simulink model "DCmotor"  (R2016a)
settings: Solver=ode23t  StartTime=0.0  StopTime=10.0  RelTol=1e-3  AbsTol=1e-3
libraries: fl_lib x12, nesl_utility x4
settings Model: Creator=STF2972  LastModifiedBy=STF2972
settings GRTTargetCC: GeneratePreprocessorConditionals=Use local settings
settings SimscapeCC: SimscapeLogType=all  SimscapeLogDataHistory=10000

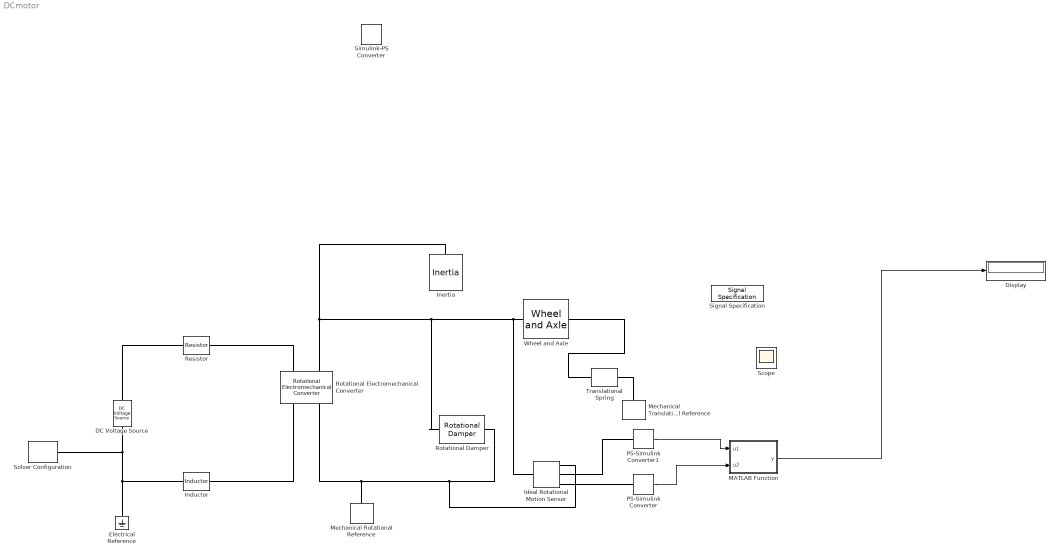
== system DCmotor ==
  DC Voltage Source : fl_lib/Electrical/Electrical Sources/DC Voltage Source  v0=5 V
  Display : Display
  Electrical Reference : fl_lib/Electrical/Electrical Elements/Electrical Reference
  Ideal Rotational Motion Sensor : fl_lib/Mechanical/Mechanical Sensors/Ideal Rotational Motion Sensor  offset=0 rad
  Inductor : fl_lib/Electrical/Electrical Elements/Inductor  l=1e-6 H  r=0 Ohm  g=1e-9 1/Ohm  i_specify=off  i_priority=None  i=0 A  v_specify=off  v_priority=None  v=0 V  i_L_specify=off  i_L_priority=High  i_L=0 A
  Inertia : fl_lib/Mechanical/Rotational Elements/Inertia  inertia=0.01 kg*m^2  w_specify=off  w_priority=High  w=0 rad/s  t_specify=off  t_priority=None  t=0 N*m
  MATLAB Function : MATLAB Function  TreatAsAtomicUnit=on
  Mechanical Rotational Reference : fl_lib/Mechanical/Rotational Elements/Mechanical Rotational Reference
  Mechanical Translational Reference : fl_lib/Mechanical/Translational Elements/Mechanical Translational Reference
  PS-Simulink Converter : nesl_utility/PS-Simulink Converter  PhysicalDomain=network_engine_domain  SubClassName=ps_output  LeftPortType=input  RightPortType=output  PseudoPeriodic=off  Frequencies=[]  Unit=deg  AffineConversion=off
  PS-Simulink Converter1 : nesl_utility/PS-Simulink Converter  PhysicalDomain=network_engine_domain  SubClassName=ps_output  LeftPortType=input  RightPortType=output  PseudoPeriodic=off  Frequencies=[]  Unit=1  AffineConversion=off
  Resistor : fl_lib/Electrical/Electrical Elements/Resistor  R=1 Ohm  i_specify=off  i_priority=None  i=0 A  v_specify=off  v_priority=None  v=0 V
  Rotational Electromechanical Converter : fl_lib/Electrical/Electrical Elements/Rotational Electromechanical Converter  K=0.1 V/(rad/s)  i_specify=off  i_priority=None  i=0 A  v_specify=off  v_priority=None  v=0 V  t_specify=off  t_priority=None  t=0 N*m  w_specify=off  w_priority=None  w=0 rad/s
  Rotational Damper : fl_lib/Mechanical/Rotational Elements/Rotational Damper  D=0.001 N*m/(rad/s)  w_specify=off  w_priority=None  w=0 rad/s  t_specify=off  t_priority=None  t=0 N*m
  Scope : Scope
  Signal Specification : SignalSpecification
  Simulink-PS Converter : nesl_utility/Simulink-PS Converter  PhysicalDomain=network_engine_domain  SubClassName=ps_input  LeftPortType=input  RightPortType=output  PseudoPeriodic=off  Frequencies=[]  NoiseDistribution=none  NoiseParameters=[]  Unit=1  AffineConversion=off  InputFiltering=off  SimscapeFilterOrder=1  InputFilterTimeConstant=0.001  UdotUserProvided=1
  Solver Configuration : nesl_utility/Solver Configuration  PhysicalDomain=network_engine_domain  SubClassName=solver  LeftPortType=input  RightPortType=generic  Accelerate=off  Tones=[]  Harmonics=[]  SimulateNoise=off  Profile=off  UseLocalSampling=off  EnableSwitchedLinearOptims=on  FrequencyDomain=off  UseCCode=off  RelTol=0.001  AbsTol=1e-06  MinStep=1e-09  ToWorkspace=off  RevertToSquareIcSolve=off  NumHomotopyIterations=100  PhasorMode=off  PhasorModeNumHarmonics=1  OverrideAbsTol=off  DoDC=on  ResidualTolerance=1e-09  UseLocalSolver=off  LocalSolverChoice=NE_BACKWARD_EULER_ADVANCER  LocalSolverSampleTime=0.001  DoFixedCost=off  MaxNonlinIter=3  MaxModeIter=2  LinearAlgebra=Sparse  DelaysMemoryBudget=1024  AutomaticFiltering=on  FilteringTimeConstant=0.001
  Translational Spring : fl_lib/Mechanical/Translational Elements/Translational Spring  spr_rate=1000 N/m  v_specify=off  v_priority=None  v=0 m/s  f_specify=off  f_priority=None  f=0 N  x_specify=off  x_priority=High  x=0 m
  Wheel and Axle : fl_lib/Mechanical/Mechanisms/Wheel and Axle  R=0.05 m  or=1  t_specify=off  t_priority=None  t=0 N*m  f_specify=off  f_priority=None  f=0 N
  wires:
  PS-Simulink Converter/1 -> MATLAB Function/2(u2)
  MATLAB Function/1(y) -> Display/1
  PS-Simulink Converter1/1 -> MATLAB Function/1(u1)
  connections:
  DC Voltage Source/LConn1 -- Resistor/LConn1
  Resistor/RConn1 -- Rotational Electromechanical Converter/LConn1
  DC Voltage Source/RConn1 -- Solver Configuration/RConn1 -- Electrical Reference/LConn1 -- Inductor/LConn1
  Inductor/RConn1 -- Rotational Electromechanical Converter/RConn1
  Rotational Electromechanical Converter/RConn2 -- Ideal Rotational Motion Sensor/RConn1 -- Rotational Damper/RConn1 -- Mechanical Rotational Reference/LConn1
  Rotational Electromechanical Converter/LConn2 -- Ideal Rotational Motion Sensor/LConn1 -- Wheel and Axle/LConn1 -- Rotational Damper/LConn1 -- Inertia/LConn1
  Translational Spring/LConn1 -- Wheel and Axle/RConn1
  Mechanical Translational Reference/LConn1 -- Translational Spring/RConn1
  Ideal Rotational Motion Sensor/RConn3 -- PS-Simulink Converter/LConn1
  Ideal Rotational Motion Sensor/RConn2 -- PS-Simulink Converter1/LConn1

== matlab function DCmotor/MATLAB Function ==
  data: u1 input; y output; u2 input
function y = fcn(u1,u2)
%#codegen
x_1=11.4591559045;
x_2 =11.4591559010;

y_1=4*10^(-10); 
y_2=-4*10^(-10); 
%%Distance measures
dist_min=0;
temp_dist=0;

c_s1 =(x_1+x_2)/2;
c_s2=(y_1+y_2)/2;

if (abs(y_1-y_2)>abs(x_1-x_2))
    rs =abs(x_1-x_2);
else 
    rs =abs(y_1-y_2);
end 

a =[c_s1 c_s2 rs];

%Until N ==m_max
N=0; % count of not self
i=0; %# of detectors


p=0.5; % default probability 
x=0; % %Selected point /occarance 
n=0; % sample size/ total number of data
m =0; % detected occurances
n_sample=10; % predefined sample size


% Detector set map(Key value pair diameter)
%detSet = containers.Map('KeyType','double','ValueType','double');
% coder.extrinsic(detset);
% detSet = java.util.Hashtable;

% Estimated coverage 99% 
%%%% Hyppthesis testing %%%%
m_max =max(5/p, 5/(1-p));
z_alpha =3.49
% Sample a point 
%%
%"x =input"
x=u1;
y =u2;
if (N<m_max) % exit criterion 
     n =n+1; % count the sample size
    if(abs (sqrt(((y-a(2))^2+(x-a(1))^2))-a(3)))>a(3)
        %%--------not-self-------
        %%                                                                                                      
        N=N+1; % count not self sample
        b=[x y abs(sqrt(((y-a(2))^2+(x-a(1))^2))-a(3))]
        if (i==0) % first detector    
            % addthe first detector to the map
            a=[a;b];  
        end 
            
      else 
            k =keys(detSet);
            temp_dist = abs (k{1}-p) ;
            key =1; % default mark of the map
            %finding the minimum distance to the point selected
            for j=1: length(k) 
                %% check if it is out 
                     temp_dist= abs (k{j}-x) ;
                    if temp_dist<dist_min
                        key =k{j}; % mark the index of the map
                        dist_min=temp_dist ; % save the smallest amount to be minimum
                    end    
            end 
            %Check if it is within the raduis of the closest detector
            %% Covered?
            if detSet(key)>dist_min
                 
                m=m+1; % count covered sample
                p =N/n; % probability of not self
                q= 1-N/n;
                z=m/sqrt(n*p*q)-sqrt(n*p/q); % evaluate z score
                if z<z_alpha % not enough coverage
                    if(N==n_sample) 
                        %% Accept all saved candidates as new detectors
                        N=0;
                        m=0;
                    else 
                        
                    end 
                else %enough coverage
                    N=m_max+1; % exist the function
                end 
            else 
                %% save the candidate
                detSet(x) = dist_min;
            end    
     end 
        
       
end 
y=a;
